simulink model "link"  (R2025b)
settings: Solver=FixedStepAuto  StartTime=0.0  StopTime=10.0  RelTol=1e-3
undefined symbols (not defined in the file): link_params, Ts_inner
settings Model: DataDictionary=project.sldd  Creator=Nick  LastModifiedBy=Rakete

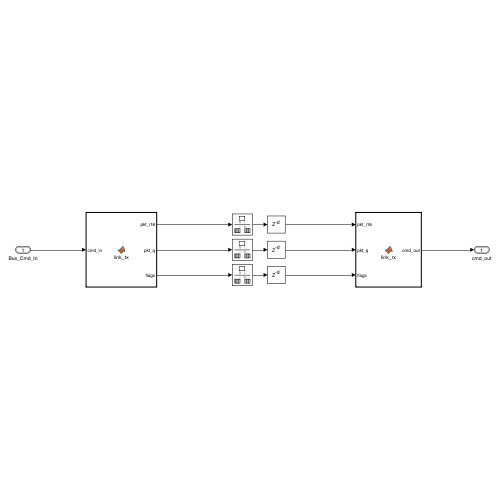
[thumbnail: Simulink's stored preview of the top-level diagram]
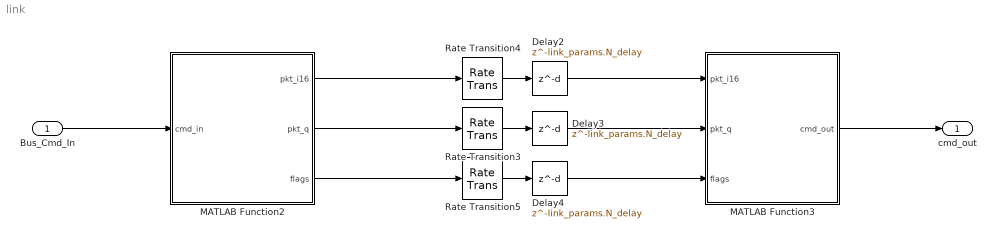
== system link ==
  Bus_Cmd_In : Inport  OutDataTypeStr=Bus: Bus_Cmd
  Delay2 : Delay  DelayLength=link_params.N_delay  InitialCondition=link_params.pkt_init_delay  SampleTime=Ts_inner
  Delay3 : Delay  DelayLength=link_params.N_delay  InitialCondition=link_params.q_init_delay  SampleTime=Ts_inner
  Delay4 : Delay  DelayLength=link_params.N_delay  InitialCondition=link_params.flags_init_delay  SampleTime=Ts_inner
  MATLAB Function2 : MATLAB Function  TreatAsAtomicUnit=on
  MATLAB Function3 : MATLAB Function  TreatAsAtomicUnit=on
  Rate Transition3 : RateTransition  OutPortSampleTime=Ts_sim
  Rate Transition4 : RateTransition  OutPortSampleTime=Ts_sim
  Rate Transition5 : RateTransition  OutPortSampleTime=Ts_sim
  cmd_out : Outport  OutDataTypeStr=Bus: Bus_Cmd
  wires:
  Rate Transition3/1 -> Delay3/1
  Rate Transition4/1 -> Delay2/1
  MATLAB Function2/1(pkt_i16) -> Rate Transition4/1
  Delay2/1 -> MATLAB Function3/1(pkt_i16)
  MATLAB Function2/2(pkt_q) -> Rate Transition3/1
  Delay3/1 -> MATLAB Function3/2(pkt_q)
  Rate Transition5/1 -> Delay4/1
  MATLAB Function2/3(flags) -> Rate Transition5/1
  Delay4/1 -> MATLAB Function3/3(flags)
  Bus_Cmd_In/1 -> MATLAB Function2/1(cmd_in)
  MATLAB Function3/1(cmd_out) -> cmd_out/1

== matlab function link/MATLAB Function2 ==
  data: cmd_in input Bus: Bus_Cmd; pkt_i16 output int16 size=[7 1]; pkt_q output uint32 size=[3 1]; flags output size=[2 1]; link_params parameter
function [pkt_i16, pkt_q, flags] = link_tx_sl(cmd_in, link_params)
%#codegen
% WRAPPER — code liegt in
% scripts\functions\link_tx.m - dieser Block ruft sie nur auf
[pkt_i16, pkt_q, flags] = link_tx(cmd_in, link_params);
end

== matlab function link/MATLAB Function3 ==
  data: pkt_i16 input int16 size=[7 1]; cmd_out output Bus: Bus_Cmd; pkt_q input uint32 size=[3 1]; flags input size=[2 1]; link_params parameter
function cmd_out = link_rx_sl(pkt_i16, pkt_q, flags, link_params)
%#codegen
% WRAPPER — code liegt in
% scripts\functions\link_rx.m - dieser Block ruft sie nur auf
cmd_out = link_rx(pkt_i16, pkt_q, flags, link_params);
end
